simulink model "system"  (R2025a)
settings: Solver=VariableStepAuto  StartTime=0.0  StopTime=10.0  RelTol=1e-3
values from neighbouring files (symbols this model uses):
  b = 0.1    [MotorspeedPIDcode.m]    (also in Params.m)
  J = 0.01    [MotorspeedPIDcode.m]    (also in Params.m)
  K = 0.01    [MotorspeedPIDcode.m]    (also in Params.m)
  L = 0.5    [MotorspeedPIDcode.m]    (also in Params.m)
  R = 1    [MotorspeedPIDcode.m]    (also in Params.m)
libraries: mpclib x1
settings Model: Creator=s4308675  LastModifiedBy=s4308675

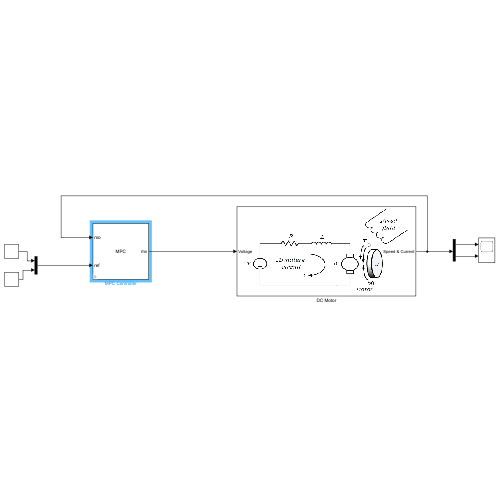
[thumbnail: Simulink's stored preview of the top-level diagram]
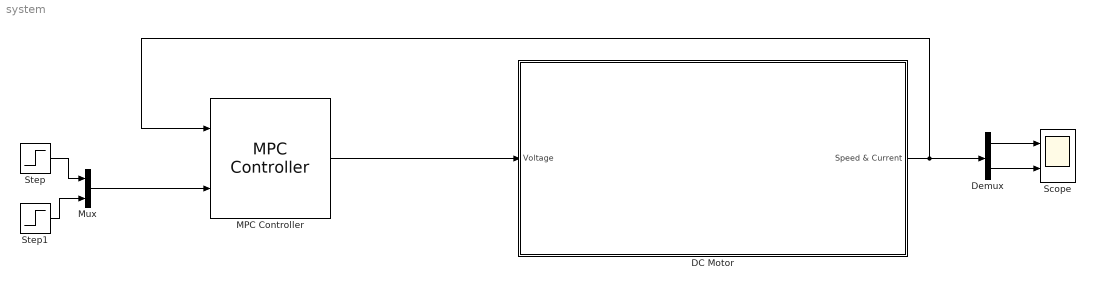
== system system ==
  DC Motor : Subsystem
      mask Display: image('Screenshot 2026-02-20 135806.png');
  Demux : Demux  Outputs=2
  MPC Controller : mpclib/MPC Controller  SCDEnableBlockLinearizationSpecification=on  is_multiple=0  enable_value=0  return_u0=off  updateMPCinCallerWorkspace=on  md_inport=off  mv_inport=off  uref_inport=off  return_cost=off  return_mvseq=off  return_qpstatus=off  return_xseq=off  return_state=off  return_ovseq=off  state_inport=off  umin_inport=off  umax_inport=off  ymin_inport=off  ymax_inport=off  cc_inport=off  ywt_inport=off  uwt_inport=off  duwt_inport=off  rhoeps_inport=off  pm_inport=off  MaximumP=10  HorizonChoice=FixedHorizon  n_ts=0.1  n_p=10  n_mv=2  n_md=1  n_ud=0  n_mo=1  n_uo=0  BlockDataType=double  SampleTimeInherited=off  switch_inport=off
  Mux : Mux  Inputs=2
  Scope : Scope  NumInputPorts=2
  Step : Step  SampleTime=0
  Step1 : Step  SampleTime=0
  wires:
  MPC Controller/1 -> DC Motor/1(Voltage)
  DC Motor/1(Speed & Current) -> Demux/1, MPC Controller/1
  Step/1 -> Mux/1
  Step1/1 -> Mux/2
  Mux/1 -> MPC Controller/2
  Demux/1 -> Scope/1
  Demux/2 -> Scope/2

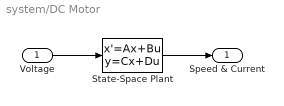
== system system/DC Motor ==
  Voltage : Inport
  State-Space Plant : StateSpace  A=[-b/J K/J; -K/L -R/L]  B=[0; 1/L]  C=[1 0]  D=0  InitialCondition=0
  Speed & Current : Outport
  wires:
  Voltage/1 -> State-Space Plant/1
  State-Space Plant/1 -> Speed & Current/1
